simulink model "QUAD1"  (R2017a)
settings: Solver=VariableStepAuto  StartTime=0.0  StopTime=10.0  RelTol=1e-3
undefined symbols (not defined in the file or in its folder): QUAD
settings Model: Creator=Dell  LastModifiedBy=Dell

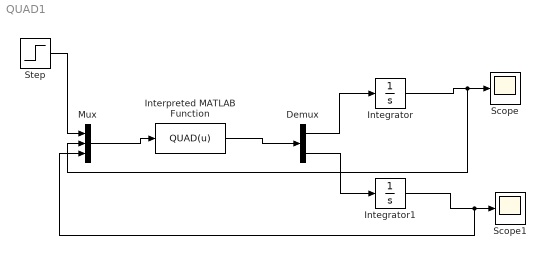
== system QUAD1 ==
  Demux : Demux  Outputs=2
  Integrator : Integrator
  Integrator1 : Integrator
  Interpreted MATLAB Function : MATLABFcn  MATLABFcn=QUAD(u)  OutputDimensions=2
  Mux : Mux  Inputs=3
  Scope : Scope
  Scope1 : Scope
  Step : Step  After=3  SampleTime=0
  wires:
  Integrator1/1 -> Scope1/1, Mux/3
  Integrator/1 -> Scope/1, Mux/2
  Demux/2 -> Integrator1/1
  Demux/1 -> Integrator/1
  Interpreted MATLAB Function/1 -> Demux/1
  Mux/1 -> Interpreted MATLAB Function/1
  Step/1 -> Mux/1
